simulink model "model2_2"  (R2013a)
settings: Solver=ode45  SolverMode=SingleTasking  StartTime=0.0  StopTime=200  FixedStep=0.01  MaxStep=0.01  MinStep=0.001  RelTol=1e-3
libraries: simulink x1
settings Model: CovMetricSettings=dwe  CovHtmlReporting=off  covSaveCumulativeToWorkspaceVar=off  CovSaveSingleToWorkspaceVar=off  CovExternalEMLEnable=on  Creator=Vjekoslav  LastModifiedBy=Vjekoslav
settings DataIOCC: LimitDataPoints=off  SaveFormat=StructureWithTime
settings DebuggingCC: UnderspecifiedInitializationDetection=Simplified  MergeDetectMultiDrivingBlocksExec=error  SolverPrmCheckMsg=none  FrameProcessingCompatibilityMsg=error  StateNameClashWarn=none  SFUnexpectedBacktrackingDiag=error  SFNoUnconditionalDefaultTransitionDiag=error
settings HardwareCC: ProdBitPerPointer=64  ProdLargestAtomicFloat=Float  ProdIntDivRoundTo=Zero  ProdEndianess=LittleEndian  ProdHWDeviceType=Specified
settings ModelReferenceCC: PropagateSignalLabelsOutOfModel=on
settings GRTTargetCC: CodeReplacementLibrary=C99 (ISO)  GeneratePreprocessorConditionals=Use local settings

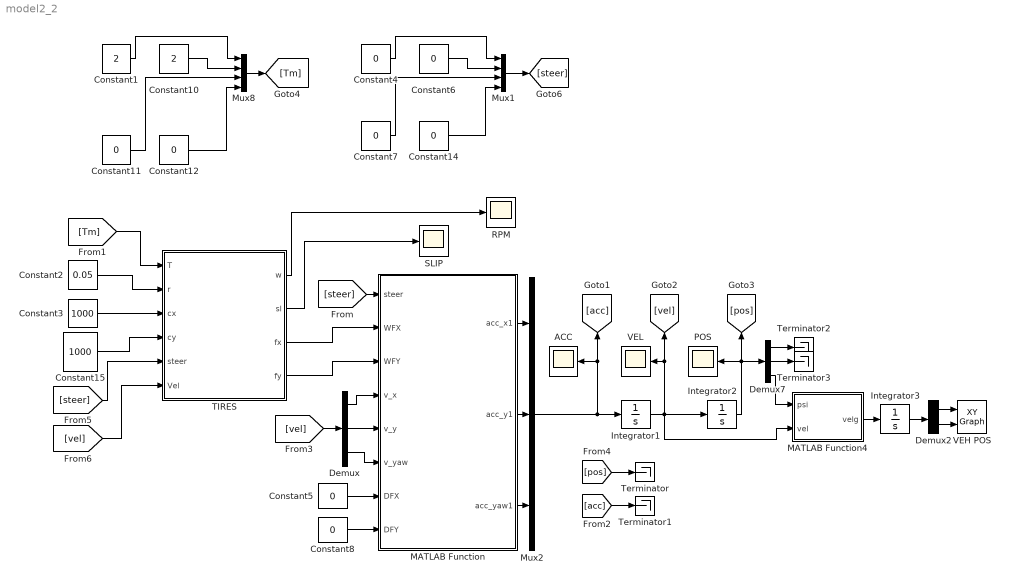
== system model2_2 ==
  ACC : Scope
      settings: TimeRange=auto  MaxDataPoints=5000  SaveToWorkspace=off  YMin=-338.87895  YMax=49.91053  SampleTime=-1
  Constant1 : Constant  Value=2
  Constant10 : Constant  Value=2
  Constant{4..8,11..12,14} (8 alike) : Constant  Value=0
  Constant15 : Constant  Value=1000
  Constant2 : Constant  Value=0.05
  Constant3 : Constant  Value=1000
  Demux : Demux  Outputs=3
  Demux2 : Demux  Outputs=2
  Demux7 : Demux  Outputs=3
  Integrator1 : Integrator  InitialCondition=[0.1 0 0]  UpperSaturationLimit=10^6  LowerSaturationLimit=-10^6  ZeroCross=off
  Integrator2 : Integrator  InitialCondition=[0 0 0]  ZeroCross=off
  Integrator3 : Integrator  InitialCondition=[0 0]  ZeroCross=off
  MATLAB Function : MATLAB Function  TreatAsAtomicUnit=on  VariantControl=Variant1
      settings: PermitHierarchicalResolution=ParametersOnly
  MATLAB Function4 : MATLAB Function  TreatAsAtomicUnit=on
      settings: PermitHierarchicalResolution=ParametersOnly
  Mux1 : Mux
  Mux2 : Mux  Inputs=3
  Mux8 : Mux
  POS : Scope
      settings: TimeRange=auto  MaxDataPoints=5000  SaveToWorkspace=off  SaveName=ScopeData  YMin=-31.74362  YMax=285.6926  SampleTime=-1
  RPM : Scope
      settings: TimeRange=auto  MaxDataPoints=5000  SaveToWorkspace=off  SaveName=ScopeData3  YMin=-43.23194  YMax=390.08746  SampleTime=-1
  SLIP : Scope
      settings: TimeRange=auto  MaxDataPoints=5000  SaveToWorkspace=off  SaveName=ScopeData4  YMin=-3.17962  YMax=0.72366  SampleTime=-1
  TIRES : Subsystem
  Terminator{,1..3} (4 alike) : Terminator
  VEH POS : simulink/Sinks/XY Graph  xmin=-50  xmax=50  ymin=-50  ymax=50  st=-1
  VEL : Scope
      settings: TimeRange=auto  MaxDataPoints=5000  SaveToWorkspace=off  SaveName=ScopeData2  YMin=-0.43037  YMax=3.85237  SampleTime=-1
  wires:
  MATLAB Function4/1(velg) -> Integrator3/1
  Demux7/3 -> MATLAB Function4/1(psi)
  Demux2/2 -> VEH POS/2
  Demux2/1 -> VEH POS/1
  MATLAB Function/3(acc_yaw1) -> Mux2/3
  Integrator3/1 -> Demux2/1
  Integrator1/1 -> MATLAB Function4/2(vel), Integrator2/1, VEL/1, [vel]
  Demux7/2 -> Terminator3/1
  Demux7/1 -> Terminator2/1
  MATLAB Function/2(acc_y1) -> Mux2/2
  MATLAB Function/1(acc_x1) -> Mux2/1
  Integrator2/1 -> Demux7/1, POS/1, [pos]
  Mux2/1 -> Integrator1/1, ACC/1, [acc]
  Constant5/1 -> MATLAB Function/7(DFX)
  Constant8/1 -> MATLAB Function/8(DFY)
  Demux/3 -> MATLAB Function/6(v_yaw)
  Demux/1 -> MATLAB Function/4(v_x)
  Demux/2 -> MATLAB Function/5(v_y)
  [vel] -> Demux/1
  [steer] -> MATLAB Function/1(steer)
  Constant12/1 -> Mux8/4
  Constant1/1 -> Mux8/1
  Constant11/1 -> Mux8/3
  Constant10/1 -> Mux8/2
  Mux8/1 -> [Tm]
  Mux1/1 -> [steer]
  Constant6/1 -> Mux1/2
  Constant7/1 -> Mux1/3
  Constant4/1 -> Mux1/1
  Constant14/1 -> Mux1/4
  [Tm] -> TIRES/1(T)
  Constant2/1 -> TIRES/2(r)
  Constant3/1 -> TIRES/3(cx)
  TIRES/4(fy) -> MATLAB Function/3(WFY)
  TIRES/3(fx) -> MATLAB Function/2(WFX)
  [steer] -> TIRES/5(steer)
  [vel] -> TIRES/6(Vel)
  TIRES/1(w) -> RPM/1
  TIRES/2(sl) -> SLIP/1
  Constant15/1 -> TIRES/4(cy)
  [pos] -> Terminator/1
  [acc] -> Terminator1/1

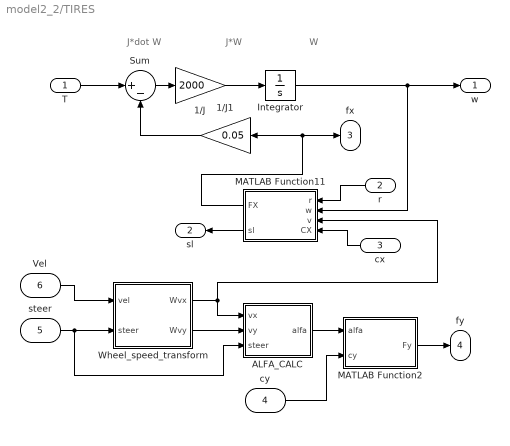
== system model2_2/TIRES ==
  note: W
  note: J*W
  note: J*dot W
  T : Inport
  r : Inport  Port=2
  cx : Inport  Port=3
  cy : Inport  Port=4
  steer : Inport  Port=5
  Vel : Inport  Port=6
  1/J : Gain  Gain=2000
  1/J1 : Gain  Gain=0.05
  ALFA_CALC : MATLAB Function  TreatAsAtomicUnit=on
      settings: PermitHierarchicalResolution=ParametersOnly
  Integrator : Integrator  InitialCondition=[0.1 0.1 0.1 0.1]  ZeroCross=off
  MATLAB Function11 : MATLAB Function  TreatAsAtomicUnit=on
      settings: PermitHierarchicalResolution=ParametersOnly
  MATLAB Function2 : MATLAB Function  TreatAsAtomicUnit=on
      settings: PermitHierarchicalResolution=ParametersOnly
  Sum : Sum  Inputs=|+-
  Wheel_speed_transform : MATLAB Function  TreatAsAtomicUnit=on
      settings: PermitHierarchicalResolution=ParametersOnly
  w : Outport
  sl : Outport  Port=2
  fx : Outport  Port=3
  fy : Outport  Port=4
  wires:
  cx/1 -> MATLAB Function11/4(CX)
  Sum/1 -> 1/J/1
  Wheel_speed_transform/1(Wvx) -> MATLAB Function11/3(v), ALFA_CALC/1(vx)
  Integrator/1 -> w/1, MATLAB Function11/2(w)
  MATLAB Function11/1(FX) -> 1/J1/1, fx/1
  T/1 -> Sum/1
  r/1 -> MATLAB Function11/1(r)
  1/J/1 -> Integrator/1
  1/J1/1 -> Sum/2
  MATLAB Function11/2(sl) -> sl/1
  Wheel_speed_transform/2(Wvy) -> ALFA_CALC/2(vy)
  ALFA_CALC/1(alfa) -> MATLAB Function2/1(alfa)
  cy/1 -> MATLAB Function2/2(cy)
  MATLAB Function2/1(Fy) -> fy/1
  steer/1 -> ALFA_CALC/3(steer), Wheel_speed_transform/2(steer)
  Vel/1 -> Wheel_speed_transform/1(vel)

== matlab function model2_2/MATLAB Function ==
  data: steer input; acc_x1 output; WFX input; WFY input; v_x input; v_y input; acc_y1 output; acc_yaw1 output; v_yaw input; DFX input; DFY input
function [acc_x1,acc_y1,acc_yaw1]= MATLAB_Function(steer,WFX,WFY,v_x,v_y,v_yaw, DFX, DFY)
%% input data
% steer steer angle of each wheel FL,FR,RL,RR [rad]
% WFX wheel force in x diretion of wheel FL,FR,RL,RR [N]
% WFY wheel force in y diretion of wheel FL,FR,RL,RR [N]
% WSS side slip of each wheel FL,FR,RL,RR [ratio]
% vehspeed vehicle speed vx,vy,yaw [m/s m/s rad/s]
% vehacc vehicle acceleraion avx,avy,ayaw [m/s^2 m/s^2 rad/s^2]
% CX tire stiffness in x dir 
% CY tire stiffness in y dir

%% vehicle data
m=12; %vehicle mass
wb=0.130; %wheel base 
lf=0.70; %front wheel track
lr=0.70; %rear wheel track
wf=0.65; % distance of cog from front track
wr=0.65; % distance of cog fron rear track
wr=0.050; %wheel radius
Arx=10; %% air resistance coefficient
Ary=10; %% air resistance coefficient

J=10; % inertial around z axis 

%% FX
Fx=cos(steer).*WFX-sin(steer).*WFY
Fy=sin(steer).*WFX+cos(steer).*WFY

Fxsum=sum(Fx)-DFX-Arx*(v_x^2)
Fysum=sum(Fy)-DFY-Ary*(v_y^2)

%% M   
M=[-wf wf -wr wr]*1/2*Fx+[lf lf -lr -lr]*Fy


%% new state
acc_x1=1/m*(Fxsum)+v_y*v_yaw;
acc_y1=1/m*(Fysum)-v_x*v_yaw;
acc_yaw1=(1/J)*M;

== matlab function model2_2/TIRES/MATLAB Function2 ==
  data: alfa input; Fy output; cy input
function Fy  = fcn(alfa,cy)
% wheel_speed=[wheel_speed wheel_speed wheel_speed wheel_speed]
% 
% sl=(wheel_rotation_speed-wheel_speed/wheel_radius)/wheel_rotation_speed[1]


alfa(find(abs(alfa)<0.01))=0;



Fy=alfa.*cy
end

== matlab function model2_2/TIRES/ALFA_CALC ==
  data: vx input; vy input; alfa output; steer input
function alfa  = alfa_calc(vx,vy,steer)
alfa=steer-atan(vy./vx);

     




end

== matlab function model2_2/MATLAB Function4 ==
  data: psi input; vel input; velg output
function velg  = fcn(psi,vel)
% wheel_speed=[wheel_speed wheel_speed wheel_speed wheel_speed]
% 
% sl=(wheel_rotation_speed-wheel_speed/wheel_radius)/wheel_rotation_speed[1]
vx=vel(1)*cos(psi)-vel(2)*sin(psi);
vy=vel(1)*sin(psi)+vel(2)*cos(psi);


velg=[vx vy]';

end

== matlab function model2_2/TIRES/Wheel_speed_transform ==
  data: vel input; Wvx output; steer input; Wvy output
function [Wvx,Wvy] = wst(vel,steer)
a=0.3;
b=0.3;
tf=0.13;
tr=0.13;
vx=vel(1);
vy=vel(2);
dpsi=vel(3);
Wangle=steer;
Wvx=[cos(Wangle(1))*(vx-tf*dpsi)+sin(Wangle(1))*(vy+a*dpsi);...
     cos(Wangle(2))*(vx+tf*dpsi)+sin(Wangle(2))*(vy+a*dpsi);...
     cos(Wangle(3))*(vx-tr*dpsi)+sin(Wangle(3))*(vy-b*dpsi);...
     cos(Wangle(4))*(vx+tr*dpsi)+sin(Wangle(4))*(vy-b*dpsi);...
     ];
Wvy=[-sin(Wangle(1))*(vx-tf*dpsi)+cos(Wangle(1))*(vy+a*dpsi);...
     -sin(Wangle(2))*(vx+tf*dpsi)+cos(Wangle(2))*(vy+a*dpsi);...
     -sin(Wangle(3))*(vx-tr*dpsi)+cos(Wangle(3))*(vy-b*dpsi);...
     -sin(Wangle(4))*(vx+tr*dpsi)+cos(Wangle(4))*(vy-b*dpsi);...
     ];




end

== matlab function model2_2/TIRES/MATLAB Function11 ==
  data: r input; FX output; w input; v input; CX input; sl output
function [FX,sl] = fcn(r,w,v,CX)
ww=r.*w(1:4);
% wheel_speed=[wheel_speed wheel_speed wheel_speed wheel_speed]
% 
% sl=(wheel_rotation_speed-wheel_speed/wheel_radius)/wheel_rotation_speed[1]

ww(find(abs(ww)<0.01))=0.01;


sa=(ww-v)./abs(w);
%sa(find(sa>1))=1;
%sa(find(sa<-1))=-1;

%sl=(-1*(u-r*2*pi*w/60))/n
sl=sa;
FX=sl*CX;
%T=-(FX)*r;
end
